simulink model "rc"  (Simulink 6.0)
settings: Solver=ode45  StartTime=0.0  StopTime=10.0  RelTol=1e-3
undefined symbols (not defined in the file): ess_cb, ess_cc, ess_coulombic_eff, ess_init_soc, ess_max_ah_cap, ess_max_volts, ess_min_volts, ess_mod_init_tmp, ess_module_num, ess_soc, ess_tmp, ess_voc, mc_min_volts, time_step
settings Model: LastModifiedBy=zhou

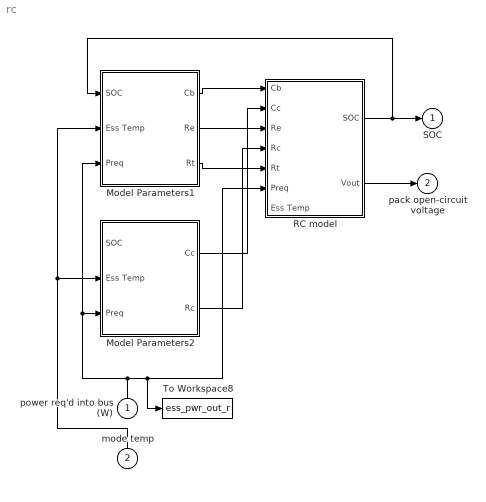
== system rc ==
  power req'd into bus (W) : Inport  Orientation=up  Port=1  LatchInput=off
  mode temp : Inport  Orientation=up  Port=2  LatchInput=off
  Model Parameters1 : Subsystem  AncestorBlock=|
      | lib_energy_storage/Ess Choices/energy
      | storage <ess>
      | RC/Model Parameters
  Model Parameters2 : Subsystem  AncestorBlock=|
      | lib_energy_storage/Ess Choices/energy
      | storage <ess>
      | RC/Model Parameters
  RC model : Subsystem  AncestorBlock=|
      | lib_energy_storage/Ess Choices/energy
      | storage <ess>
      | RC/RC model
  To Workspace8 : ToWorkspace  VariableName=ess_pwr_out_r  SampleTime=-1  SaveFormat=Array
  SOC : Outport  InitialOutput=0
  pack open-circuit voltage : Outport  Port=2  InitialOutput=0
  wires:
  Model Parameters1/1(Cb) -> RC model/1(Cb)
  Model Parameters1/2(Re) -> RC model/3(Re)
  Model Parameters1/3(Rt) -> RC model/5(Rt)
  power req'd into bus (W)/1 -> RC model/6(Preq), To Workspace8/1, Model Parameters1/3(Preq), Model Parameters2/3(Preq)
  Model Parameters2/1(Cc) -> RC model/2(Cc)
  Model Parameters2/2(Rc) -> RC model/4(Rc)
  mode temp/1 -> Model Parameters1/2(Ess Temp), Model Parameters2/2(Ess Temp)
  RC model/2(Vout) -> pack open-circuit voltage/1
  RC model/1(SOC) -> SOC/1, Model Parameters1/1(SOC)

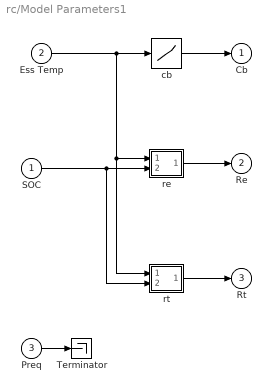
== system rc/Model Parameters1 ==
  SOC : Inport  Port=1  LatchInput=off
  Ess Temp : Inport  Port=2  LatchInput=off
  Preq : Inport  Port=3  LatchInput=off
  Terminator : Terminator
  cb : Lookup  DialogController=Simulink.DDGSource  InputValues=ess_tmp  OutputValues=ess_cb  SaturateOnIntegerOverflow=on
  re : Subsystem  mask(2-D Table Lookup){@1=ess_tmp, @2=ess_soc, @3=ess_re}
      mask prompts: @1 "X Index"; @2 "Y Index"; @3 "Table"
      mask help:
      | Two Dimensional Table Lookup
      | The first input corresponds to X Index and the second input corresponds to the Y Index
      mask init:
      | xindex=@1; yindex=@2; table=@3; sftab2chk(xindex,yindex,table);
      mask Help: This block returns a linearly interpolated intersection from the table using the X index (which corresponds to the rows of the table) and the Y index (which corresponds to the columns of the table).  Extrapolation is used.
      mask Display: plot(-10,-10,110,110,[90,50,10],[90,40,30],[90,50,10],[50,26,20],[90,50,10],[22,13,10])
  rt : Subsystem  mask(2-D Table Lookup){@1=ess_tmp, @2=ess_soc, @3=ess_rt}
      mask prompts: @1 "X Index"; @2 "Y Index"; @3 "Table"
      mask help:
      | Two Dimensional Table Lookup
      | The first input corresponds to X Index and the second input corresponds to the Y Index
      mask init:
      | xindex=@1; yindex=@2; table=@3; sftab2chk(xindex,yindex,table);
      mask Help: This block returns a linearly interpolated intersection from the table using the X index (which corresponds to the rows of the table) and the Y index (which corresponds to the columns of the table).  Extrapolation is used.
      mask Display: plot(-10,-10,110,110,[90,50,10],[90,40,30],[90,50,10],[50,26,20],[90,50,10],[22,13,10])
  Cb : Outport  InitialOutput=0
  Re : Outport  Port=2  InitialOutput=0
  Rt : Outport  Port=3  InitialOutput=0
  wires:
  Ess Temp/1 -> cb/1, re/1(x0), rt/1(x0)
  Preq/1 -> Terminator/1
  SOC/1 -> re/2(y0), rt/2(y0)
  cb/1 -> Cb/1
  rt/1(table out) -> Rt/1
  re/1(table out) -> Re/1

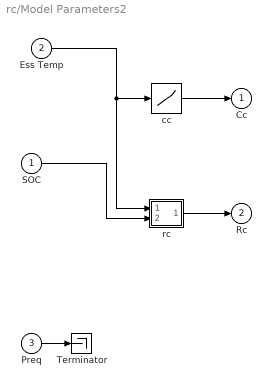
== system rc/Model Parameters2 ==
  SOC : Inport  Port=1  LatchInput=off
  Ess Temp : Inport  Port=2  LatchInput=off
  Preq : Inport  Port=3  LatchInput=off
  Terminator : Terminator
  cc : Lookup  DialogController=Simulink.DDGSource  InputValues=ess_tmp  OutputValues=ess_cc  SaturateOnIntegerOverflow=on
  rc : Subsystem  mask(2-D Table Lookup){@1=ess_tmp, @2=ess_soc, @3=ess_rc}
      mask prompts: @1 "X Index"; @2 "Y Index"; @3 "Table"
      mask help:
      | Two Dimensional Table Lookup
      | The first input corresponds to X Index and the second input corresponds to the Y Index
      mask init:
      | xindex=@1; yindex=@2; table=@3; sftab2chk(xindex,yindex,table);
      mask Help: This block returns a linearly interpolated intersection from the table using the X index (which corresponds to the rows of the table) and the Y index (which corresponds to the columns of the table).  Extrapolation is used.
      mask Display: plot(-10,-10,110,110,[90,50,10],[90,40,30],[90,50,10],[50,26,20],[90,50,10],[22,13,10])
  Cc : Outport  InitialOutput=0
  Rc : Outport  Port=2  InitialOutput=0
  wires:
  Ess Temp/1 -> cc/1, rc/1(x0)
  Preq/1 -> Terminator/1
  SOC/1 -> rc/2(y0)
  cc/1 -> Cc/1
  rc/1(table out) -> Rc/1

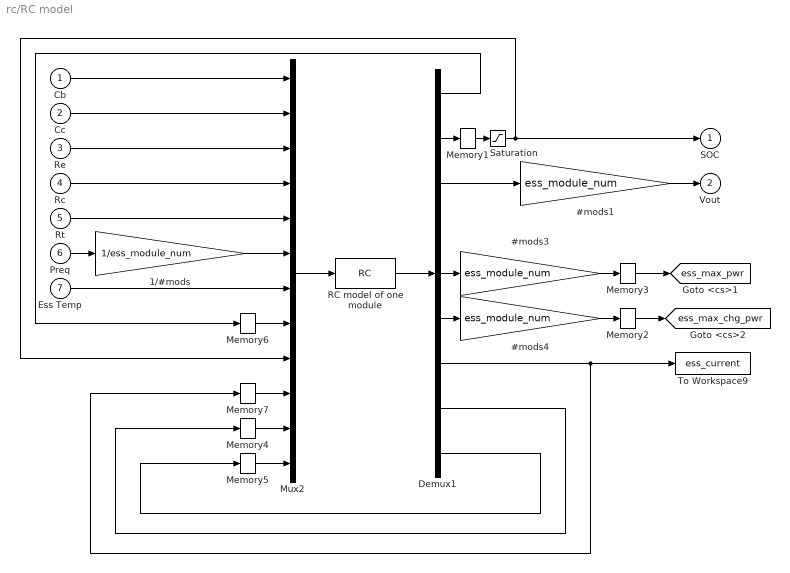
== system rc/RC model ==
  Cb : Inport  Port=1  LatchInput=off
  Cc : Inport  Port=2  LatchInput=off
  Re : Inport  Port=3  LatchInput=off
  Rc : Inport  Port=4  LatchInput=off
  Rt : Inport  Port=5  LatchInput=off
  Preq : Inport  Port=6  LatchInput=off
  Ess Temp : Inport  Port=7  LatchInput=off
  #mods1 : Gain  Gain=ess_module_num  SaturateOnIntegerOverflow=on
  #mods3 : Gain  Gain=ess_module_num  SaturateOnIntegerOverflow=on
  #mods4 : Gain  Gain=ess_module_num  SaturateOnIntegerOverflow=on
  1/#mods : Gain  Gain=1/ess_module_num  SaturateOnIntegerOverflow=on
  Demux1 : Demux  Outputs=9
  Memory1 : Memory  X0=ess_init_soc
  Memory{2..3,6..7} (4 alike) : Memory
  Memory4 : Memory  X0=ess_init_soc
  Memory5 : Memory  X0=-1
  Mux2 : Mux  Inputs=12
  RC model of one module : S-Function  FunctionName=RC  Parameters=ess_min_volts,ess_max_volts,mc_min_volts/ess_module_num,ess_soc,ess_tmp,ess_voc,ess_init_soc,ess_mod_init_tmp,ess_max_ah_cap,time_step,ess_coulombic_eff
  Saturation : Saturate  UpperLimit=1  LowerLimit=0
  To Workspace9 : ToWorkspace  VariableName=ess_current  SampleTime=-1  SaveFormat=Array
  SOC : Outport  InitialOutput=0
  Vout : Outport  Port=2  InitialOutput=0
  tag scope: ess_max_chg_pwr=global, ess_max_pwr=global
  wires:
  Saturation/1 -> SOC/1, Mux2/9
  RC model of one module/1 -> Demux1/1
  #mods1/1 -> Vout/1
  Demux1/3 -> #mods1/1
  Demux1/1 -> Memory6/1
  1/#mods/1 -> Mux2/6
  Preq/1 -> 1/#mods/1
  Mux2/1 -> RC model of one module/1
  Rt/1 -> Mux2/5
  Rc/1 -> Mux2/4
  Re/1 -> Mux2/3
  Cc/1 -> Mux2/2
  Cb/1 -> Mux2/1
  Ess Temp/1 -> Mux2/7
  Demux1/7 -> To Workspace9/1, Memory7/1
  Demux1/6 -> #mods4/1
  Memory2/1 -> [ess_max_chg_pwr]
  Demux1/5 -> #mods3/1
  Memory3/1 -> [ess_max_pwr]
  Demux1/2 -> Memory1/1
  Demux1/8 -> Memory4/1
  Demux1/9 -> Memory5/1
  Memory6/1 -> Mux2/8
  Memory7/1 -> Mux2/10
  Memory4/1 -> Mux2/11
  Memory5/1 -> Mux2/12
  Memory1/1 -> Saturation/1
  #mods3/1 -> Memory3/1
  #mods4/1 -> Memory2/1

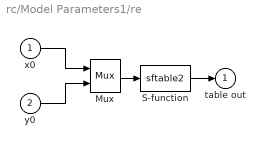
== system rc/Model Parameters1/re ==
  x0 : Inport  Port=1  LatchInput=off
  y0 : Inport  Port=2  LatchInput=off
  Mux : Mux  Inputs=2
  S-function : S-Function  FunctionName=sftable2  Parameters=xindex, yindex, table
  table out : Outport  InitialOutput=0
  wires:
  y0/1 -> Mux/2
  S-function/1 -> table out/1
  x0/1 -> Mux/1
  Mux/1 -> S-function/1

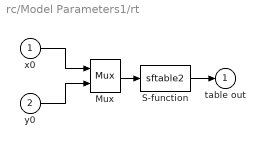
== system rc/Model Parameters1/rt ==
  x0 : Inport  Port=1  LatchInput=off
  y0 : Inport  Port=2  LatchInput=off
  Mux : Mux  Inputs=2
  S-function : S-Function  FunctionName=sftable2  Parameters=xindex, yindex, table
  table out : Outport  InitialOutput=0
  wires:
  y0/1 -> Mux/2
  S-function/1 -> table out/1
  x0/1 -> Mux/1
  Mux/1 -> S-function/1

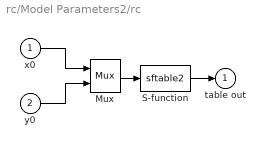
== system rc/Model Parameters2/rc ==
  x0 : Inport  Port=1  LatchInput=off
  y0 : Inport  Port=2  LatchInput=off
  Mux : Mux  Inputs=2
  S-function : S-Function  FunctionName=sftable2  Parameters=xindex, yindex, table
  table out : Outport  InitialOutput=0
  wires:
  Mux/1 -> S-function/1
  x0/1 -> Mux/1
  S-function/1 -> table out/1
  y0/1 -> Mux/2
